simulink model "ControlDes"  (R2026a)
settings: Solver=ode3  StopTime=4  FixedStep=0.001  EnableMultiTasking=on
(part 12 of 12)

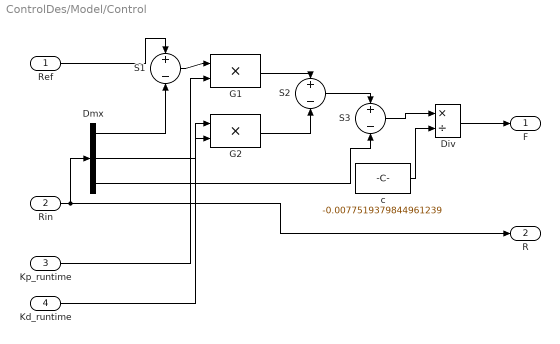
== system ControlDes/Model/Control ==
  Ref : Inport
  Rin : Inport  Port=2
  Kp_runtime : Inport  Port=3  OutDataTypeStr=double
  Kd_runtime : Inport  Port=4  OutDataTypeStr=double
  Div : Product  Inputs=*/
  Dmx : Demux  Outputs=3
  G1 : Product  Inputs=**
  G2 : Product  Inputs=**
  S1 : Sum  Inputs=+-
  S2 : Sum  Inputs=+-
  S3 : Sum  Inputs=+-
  c : Constant  Value=-0.0077519379844961239
  F : Outport
  R : Outport  Port=2
  wires:
  Div/1 -> F/1
  c/1 -> Div/2
  S3/1 -> Div/1
  Dmx/3 -> S3/2
  S2/1 -> S3/1
  G2/1 -> S2/2
  G1/1 -> S2/1
  Dmx/2 -> G2/1
  S1/1 -> G1/1
  Dmx/1 -> S1/2
  Rin/1 -> R/1, Dmx/1
  Ref/1 -> S1/1
  Kp_runtime/1 -> G1/2
  Kd_runtime/1 -> G2/2

== system ControlDes/Model/Matriz ==
  u : Inport
  A_eso_runtime : Inport  Port=2  OutDataTypeStr=double  PortDimensions=[3 3]
  B_eso_runtime : Inport  Port=3  OutDataTypeStr=double  PortDimensions=[3 2]
  C_eso_runtime : Inport  Port=4  OutDataTypeStr=double  PortDimensions=[3 3]
  D_eso_runtime : Inport  Port=5  OutDataTypeStr=double  PortDimensions=[3 2]
  A : Product  Inputs=**  Multiplication=Matrix(*)
  B : Product  Inputs=**  Multiplication=Matrix(*)
  C : Product  Inputs=**  Multiplication=Matrix(*)
  D : Product  Inputs=**  Multiplication=Matrix(*)
  State : UnitDelay  InitialCondition=[0.009;0;0]  SampleTime=0.001
  SumX : Sum
  SumY : Sum
  y : Outport
  wires:
  SumY/1 -> y/1
  D/1 -> SumY/2
  C/1 -> SumY/1
  State/1 -> A/2, C/2
  SumX/1 -> State/1
  B/1 -> SumX/2
  A/1 -> SumX/1
  u/1 -> B/2, D/2
  A_eso_runtime/1 -> A/1
  B_eso_runtime/1 -> B/1
  C_eso_runtime/1 -> C/1
  D_eso_runtime/1 -> D/1

== system ControlDes/Model1/Control ==
  Ref : Inport
  Rin : Inport  Port=2
  Kp_runtime : Inport  Port=3  OutDataTypeStr=double
  Kd_runtime : Inport  Port=4  OutDataTypeStr=double
  Div : Product  Inputs=*/
  Dmx : Demux  Outputs=3
  G1 : Product  Inputs=**
  G2 : Product  Inputs=**
  S1 : Sum  Inputs=+-
  S2 : Sum  Inputs=+-
  S3 : Sum  Inputs=+-
  c : Constant  Value=-0.010335917312661499
  F : Outport
  R : Outport  Port=2
  wires:
  Div/1 -> F/1
  c/1 -> Div/2
  S3/1 -> Div/1
  Dmx/3 -> S3/2
  S2/1 -> S3/1
  G2/1 -> S2/2
  G1/1 -> S2/1
  Dmx/2 -> G2/1
  S1/1 -> G1/1
  Dmx/1 -> S1/2
  Rin/1 -> R/1, Dmx/1
  Ref/1 -> S1/1
  Kp_runtime/1 -> G1/2
  Kd_runtime/1 -> G2/2

== system ControlDes/Model1/Matriz ==
  u : Inport
  A_eso_runtime : Inport  Port=2  OutDataTypeStr=double  PortDimensions=[3 3]
  B_eso_runtime : Inport  Port=3  OutDataTypeStr=double  PortDimensions=[3 2]
  C_eso_runtime : Inport  Port=4  OutDataTypeStr=double  PortDimensions=[3 3]
  D_eso_runtime : Inport  Port=5  OutDataTypeStr=double  PortDimensions=[3 2]
  A : Product  Inputs=**  Multiplication=Matrix(*)
  B : Product  Inputs=**  Multiplication=Matrix(*)
  C : Product  Inputs=**  Multiplication=Matrix(*)
  D : Product  Inputs=**  Multiplication=Matrix(*)
  State : UnitDelay  InitialCondition=[0.018;0;9.8]  SampleTime=0.001
  SumX : Sum
  SumY : Sum
  y : Outport
  wires:
  SumY/1 -> y/1
  D/1 -> SumY/2
  C/1 -> SumY/1
  State/1 -> A/2, C/2
  SumX/1 -> State/1
  B/1 -> SumX/2
  A/1 -> SumX/1
  u/1 -> B/2, D/2
  A_eso_runtime/1 -> A/1
  B_eso_runtime/1 -> B/1
  C_eso_runtime/1 -> C/1
  D_eso_runtime/1 -> D/1

== system ControlDes/Model2/Control ==
  Ref : Inport
  Rin : Inport  Port=2
  Kp_runtime : Inport  Port=3  OutDataTypeStr=double
  Kd_runtime : Inport  Port=4  OutDataTypeStr=double
  Div : Product  Inputs=*/
  Dmx : Demux  Outputs=3
  G1 : Product  Inputs=**
  G2 : Product  Inputs=**
  S1 : Sum  Inputs=+-
  S2 : Sum  Inputs=+-
  S3 : Sum  Inputs=+-
  c : Constant  Value=-0.010335917312661499
  F : Outport
  R : Outport  Port=2
  wires:
  Div/1 -> F/1
  c/1 -> Div/2
  S3/1 -> Div/1
  Dmx/3 -> S3/2
  S2/1 -> S3/1
  G2/1 -> S2/2
  G1/1 -> S2/1
  Dmx/2 -> G2/1
  S1/1 -> G1/1
  Dmx/1 -> S1/2
  Rin/1 -> R/1, Dmx/1
  Ref/1 -> S1/1
  Kp_runtime/1 -> G1/2
  Kd_runtime/1 -> G2/2

== system ControlDes/Model2/Matriz ==
  u : Inport
  A_eso_runtime : Inport  Port=2  OutDataTypeStr=double  PortDimensions=[3 3]
  B_eso_runtime : Inport  Port=3  OutDataTypeStr=double  PortDimensions=[3 2]
  C_eso_runtime : Inport  Port=4  OutDataTypeStr=double  PortDimensions=[3 3]
  D_eso_runtime : Inport  Port=5  OutDataTypeStr=double  PortDimensions=[3 2]
  A : Product  Inputs=**  Multiplication=Matrix(*)
  B : Product  Inputs=**  Multiplication=Matrix(*)
  C : Product  Inputs=**  Multiplication=Matrix(*)
  D : Product  Inputs=**  Multiplication=Matrix(*)
  State : UnitDelay  InitialCondition=[0.018;0;9.8]  SampleTime=0.001
  SumX : Sum
  SumY : Sum
  y : Outport
  wires:
  SumY/1 -> y/1
  D/1 -> SumY/2
  C/1 -> SumY/1
  State/1 -> A/2, C/2
  SumX/1 -> State/1
  B/1 -> SumX/2
  A/1 -> SumX/1
  u/1 -> B/2, D/2
  A_eso_runtime/1 -> A/1
  B_eso_runtime/1 -> B/1
  C_eso_runtime/1 -> C/1
  D_eso_runtime/1 -> D/1

== system ControlDes/Model3/Control ==
  Ref : Inport
  Rin : Inport  Port=2
  Kp_runtime : Inport  Port=3  OutDataTypeStr=double
  Kd_runtime : Inport  Port=4  OutDataTypeStr=double
  Div : Product  Inputs=*/
  Dmx : Demux  Outputs=3
  G1 : Product  Inputs=**
  G2 : Product  Inputs=**
  S1 : Sum  Inputs=+-
  S2 : Sum  Inputs=+-
  S3 : Sum  Inputs=+-
  c : Constant  Value=-0.010335917312661499
  F : Outport
  wires:
  Div/1 -> F/1
  c/1 -> Div/2
  S3/1 -> Div/1
  Dmx/3 -> S3/2
  S2/1 -> S3/1
  G2/1 -> S2/2
  G1/1 -> S2/1
  Dmx/2 -> G2/1
  S1/1 -> G1/1
  Dmx/1 -> S1/2
  Rin/1 -> Dmx/1
  Ref/1 -> S1/1
  Kp_runtime/1 -> G1/2
  Kd_runtime/1 -> G2/2

== system ControlDes/Model3/Matriz ==
  u : Inport
  A_eso_runtime : Inport  Port=2  OutDataTypeStr=double  PortDimensions=[3 3]
  B_eso_runtime : Inport  Port=3  OutDataTypeStr=double  PortDimensions=[3 2]
  C_eso_runtime : Inport  Port=4  OutDataTypeStr=double  PortDimensions=[3 3]
  D_eso_runtime : Inport  Port=5  OutDataTypeStr=double  PortDimensions=[3 2]
  A : Product  Inputs=**  Multiplication=Matrix(*)
  B : Product  Inputs=**  Multiplication=Matrix(*)
  C : Product  Inputs=**  Multiplication=Matrix(*)
  D : Product  Inputs=**  Multiplication=Matrix(*)
  State : UnitDelay  InitialCondition=[0.018;0;9.8]  SampleTime=0.001
  SumX : Sum
  SumY : Sum
  y : Outport
  wires:
  SumY/1 -> y/1
  D/1 -> SumY/2
  C/1 -> SumY/1
  State/1 -> A/2, C/2
  SumX/1 -> State/1
  B/1 -> SumX/2
  A/1 -> SumX/1
  u/1 -> B/2, D/2
  A_eso_runtime/1 -> A/1
  B_eso_runtime/1 -> B/1
  C_eso_runtime/1 -> C/1
  D_eso_runtime/1 -> D/1

== system ControlDes/Model4/Control ==
  Ref : Inport
  Rin : Inport  Port=2
  Kp_runtime : Inport  Port=3  OutDataTypeStr=double
  Kd_runtime : Inport  Port=4  OutDataTypeStr=double
  Div : Product  Inputs=*/
  Dmx : Demux  Outputs=3
  G1 : Product  Inputs=**
  G2 : Product  Inputs=**
  S1 : Sum  Inputs=+-
  S2 : Sum  Inputs=+-
  S3 : Sum  Inputs=+-
  c : Constant  Value=-0.0077519379844961239
  F : Outport
  R : Outport  Port=2
  wires:
  Div/1 -> F/1
  c/1 -> Div/2
  S3/1 -> Div/1
  Dmx/3 -> S3/2
  S2/1 -> S3/1
  G2/1 -> S2/2
  G1/1 -> S2/1
  Dmx/2 -> G2/1
  S1/1 -> G1/1
  Dmx/1 -> S1/2
  Rin/1 -> R/1, Dmx/1
  Ref/1 -> S1/1
  Kp_runtime/1 -> G1/2
  Kd_runtime/1 -> G2/2

== system ControlDes/Model4/Matriz ==
  u : Inport
  A_eso_runtime : Inport  Port=2  OutDataTypeStr=double  PortDimensions=[3 3]
  B_eso_runtime : Inport  Port=3  OutDataTypeStr=double  PortDimensions=[3 2]
  C_eso_runtime : Inport  Port=4  OutDataTypeStr=double  PortDimensions=[3 3]
  D_eso_runtime : Inport  Port=5  OutDataTypeStr=double  PortDimensions=[3 2]
  A : Product  Inputs=**  Multiplication=Matrix(*)
  B : Product  Inputs=**  Multiplication=Matrix(*)
  C : Product  Inputs=**  Multiplication=Matrix(*)
  D : Product  Inputs=**  Multiplication=Matrix(*)
  State : UnitDelay  InitialCondition=[0.01023;0;0]  SampleTime=0.001
  SumX : Sum
  SumY : Sum
  y : Outport
  wires:
  SumY/1 -> y/1
  D/1 -> SumY/2
  C/1 -> SumY/1
  State/1 -> A/2, C/2
  SumX/1 -> State/1
  B/1 -> SumX/2
  A/1 -> SumX/1
  u/1 -> B/2, D/2
  A_eso_runtime/1 -> A/1
  B_eso_runtime/1 -> B/1
  C_eso_runtime/1 -> C/1
  D_eso_runtime/1 -> D/1

== system ControlDes/Model5/Control ==
  Ref : Inport
  Rin : Inport  Port=2
  Kp_runtime : Inport  Port=3  OutDataTypeStr=double
  Kd_runtime : Inport  Port=4  OutDataTypeStr=double
  Div : Product  Inputs=*/
  Dmx : Demux  Outputs=3
  G1 : Product  Inputs=**
  G2 : Product  Inputs=**
  S1 : Sum  Inputs=+-
  S2 : Sum  Inputs=+-
  S3 : Sum  Inputs=+-
  c : Constant  Value=-0.010335917312661499
  F : Outport
  R : Outport  Port=2
  wires:
  Div/1 -> F/1
  c/1 -> Div/2
  S3/1 -> Div/1
  Dmx/3 -> S3/2
  S2/1 -> S3/1
  G2/1 -> S2/2
  G1/1 -> S2/1
  Dmx/2 -> G2/1
  S1/1 -> G1/1
  Dmx/1 -> S1/2
  Rin/1 -> R/1, Dmx/1
  Ref/1 -> S1/1
  Kp_runtime/1 -> G1/2
  Kd_runtime/1 -> G2/2

== system ControlDes/Model5/Matriz ==
  u : Inport
  A_eso_runtime : Inport  Port=2  OutDataTypeStr=double  PortDimensions=[3 3]
  B_eso_runtime : Inport  Port=3  OutDataTypeStr=double  PortDimensions=[3 2]
  C_eso_runtime : Inport  Port=4  OutDataTypeStr=double  PortDimensions=[3 3]
  D_eso_runtime : Inport  Port=5  OutDataTypeStr=double  PortDimensions=[3 2]
  A : Product  Inputs=**  Multiplication=Matrix(*)
  B : Product  Inputs=**  Multiplication=Matrix(*)
  C : Product  Inputs=**  Multiplication=Matrix(*)
  D : Product  Inputs=**  Multiplication=Matrix(*)
  State : UnitDelay  InitialCondition=[0.018;0;9.8]  SampleTime=0.001
  SumX : Sum
  SumY : Sum
  y : Outport
  wires:
  SumY/1 -> y/1
  D/1 -> SumY/2
  C/1 -> SumY/1
  State/1 -> A/2, C/2
  SumX/1 -> State/1
  B/1 -> SumX/2
  A/1 -> SumX/1
  u/1 -> B/2, D/2
  A_eso_runtime/1 -> A/1
  B_eso_runtime/1 -> B/1
  C_eso_runtime/1 -> C/1
  D_eso_runtime/1 -> D/1

== system ControlDes/Model6/Control ==
  Ref : Inport
  Rin : Inport  Port=2
  Kp_runtime : Inport  Port=3  OutDataTypeStr=double
  Kd_runtime : Inport  Port=4  OutDataTypeStr=double
  Div : Product  Inputs=*/
  Dmx : Demux  Outputs=3
  G1 : Product  Inputs=**
  G2 : Product  Inputs=**
  S1 : Sum  Inputs=+-
  S2 : Sum  Inputs=+-
  S3 : Sum  Inputs=+-
  c : Constant  Value=-0.0077519379844961239
  F : Outport
  R : Outport  Port=2
  wires:
  Div/1 -> F/1
  c/1 -> Div/2
  S3/1 -> Div/1
  Dmx/3 -> S3/2
  S2/1 -> S3/1
  G2/1 -> S2/2
  G1/1 -> S2/1
  Dmx/2 -> G2/1
  S1/1 -> G1/1
  Dmx/1 -> S1/2
  Rin/1 -> R/1, Dmx/1
  Ref/1 -> S1/1
  Kp_runtime/1 -> G1/2
  Kd_runtime/1 -> G2/2

== system ControlDes/Model6/Matriz ==
  u : Inport
  A_eso_runtime : Inport  Port=2  OutDataTypeStr=double  PortDimensions=[3 3]
  B_eso_runtime : Inport  Port=3  OutDataTypeStr=double  PortDimensions=[3 2]
  C_eso_runtime : Inport  Port=4  OutDataTypeStr=double  PortDimensions=[3 3]
  D_eso_runtime : Inport  Port=5  OutDataTypeStr=double  PortDimensions=[3 2]
  A : Product  Inputs=**  Multiplication=Matrix(*)
  B : Product  Inputs=**  Multiplication=Matrix(*)
  C : Product  Inputs=**  Multiplication=Matrix(*)
  D : Product  Inputs=**  Multiplication=Matrix(*)
  State : UnitDelay  InitialCondition=[0.009;0;0]  SampleTime=0.001
  SumX : Sum
  SumY : Sum
  y : Outport
  wires:
  SumY/1 -> y/1
  D/1 -> SumY/2
  C/1 -> SumY/1
  State/1 -> A/2, C/2
  SumX/1 -> State/1
  B/1 -> SumX/2
  A/1 -> SumX/1
  u/1 -> B/2, D/2
  A_eso_runtime/1 -> A/1
  B_eso_runtime/1 -> B/1
  C_eso_runtime/1 -> C/1
  D_eso_runtime/1 -> D/1

== system ControlDes/Model7/Control ==
  Ref : Inport
  Rin : Inport  Port=2
  Kp_runtime : Inport  Port=3  OutDataTypeStr=double
  Kd_runtime : Inport  Port=4  OutDataTypeStr=double
  Div : Product  Inputs=*/
  Dmx : Demux  Outputs=3
  G1 : Product  Inputs=**
  G2 : Product  Inputs=**
  S1 : Sum  Inputs=+-
  S2 : Sum  Inputs=+-
  S3 : Sum  Inputs=+-
  c : Constant  Value=-0.0077519379844961239
  F : Outport
  R : Outport  Port=2
  wires:
  Div/1 -> F/1
  c/1 -> Div/2
  S3/1 -> Div/1
  Dmx/3 -> S3/2
  S2/1 -> S3/1
  G2/1 -> S2/2
  G1/1 -> S2/1
  Dmx/2 -> G2/1
  S1/1 -> G1/1
  Dmx/1 -> S1/2
  Rin/1 -> R/1, Dmx/1
  Ref/1 -> S1/1
  Kp_runtime/1 -> G1/2
  Kd_runtime/1 -> G2/2

== system ControlDes/Model7/Matriz ==
  u : Inport
  A_eso_runtime : Inport  Port=2  OutDataTypeStr=double  PortDimensions=[3 3]
  B_eso_runtime : Inport  Port=3  OutDataTypeStr=double  PortDimensions=[3 2]
  C_eso_runtime : Inport  Port=4  OutDataTypeStr=double  PortDimensions=[3 3]
  D_eso_runtime : Inport  Port=5  OutDataTypeStr=double  PortDimensions=[3 2]
  A : Product  Inputs=**  Multiplication=Matrix(*)
  B : Product  Inputs=**  Multiplication=Matrix(*)
  C : Product  Inputs=**  Multiplication=Matrix(*)
  D : Product  Inputs=**  Multiplication=Matrix(*)
  State : UnitDelay  InitialCondition=[0.01023;0;0]  SampleTime=0.001
  SumX : Sum
  SumY : Sum
  y : Outport
  wires:
  SumY/1 -> y/1
  D/1 -> SumY/2
  C/1 -> SumY/1
  State/1 -> A/2, C/2
  SumX/1 -> State/1
  B/1 -> SumX/2
  A/1 -> SumX/1
  u/1 -> B/2, D/2
  A_eso_runtime/1 -> A/1
  B_eso_runtime/1 -> B/1
  C_eso_runtime/1 -> C/1
  D_eso_runtime/1 -> D/1

== system ControlDes/Model8/Control ==
  Ref : Inport
  Rin : Inport  Port=2
  Kp_runtime : Inport  Port=3  OutDataTypeStr=double
  Kd_runtime : Inport  Port=4  OutDataTypeStr=double
  Div : Product  Inputs=*/
  Dmx : Demux  Outputs=3
  G1 : Product  Inputs=**
  G2 : Product  Inputs=**
  S1 : Sum  Inputs=+-
  S2 : Sum  Inputs=+-
  S3 : Sum  Inputs=+-
  c : Constant  Value=-0.0077519379844961239
  F : Outport
  R : Outport  Port=2
  wires:
  Div/1 -> F/1
  c/1 -> Div/2
  S3/1 -> Div/1
  Dmx/3 -> S3/2
  S2/1 -> S3/1
  G2/1 -> S2/2
  G1/1 -> S2/1
  Dmx/2 -> G2/1
  S1/1 -> G1/1
  Dmx/1 -> S1/2
  Rin/1 -> R/1, Dmx/1
  Ref/1 -> S1/1
  Kp_runtime/1 -> G1/2
  Kd_runtime/1 -> G2/2

== system ControlDes/Model8/Matriz ==
  u : Inport
  A_eso_runtime : Inport  Port=2  OutDataTypeStr=double  PortDimensions=[3 3]
  B_eso_runtime : Inport  Port=3  OutDataTypeStr=double  PortDimensions=[3 2]
  C_eso_runtime : Inport  Port=4  OutDataTypeStr=double  PortDimensions=[3 3]
  D_eso_runtime : Inport  Port=5  OutDataTypeStr=double  PortDimensions=[3 2]
  A : Product  Inputs=**  Multiplication=Matrix(*)
  B : Product  Inputs=**  Multiplication=Matrix(*)
  C : Product  Inputs=**  Multiplication=Matrix(*)
  D : Product  Inputs=**  Multiplication=Matrix(*)
  State : UnitDelay  InitialCondition=[0.009;0;0]  SampleTime=0.001
  SumX : Sum
  SumY : Sum
  y : Outport
  wires:
  SumY/1 -> y/1
  D/1 -> SumY/2
  C/1 -> SumY/1
  State/1 -> A/2, C/2
  SumX/1 -> State/1
  B/1 -> SumX/2
  A/1 -> SumX/1
  u/1 -> B/2, D/2
  A_eso_runtime/1 -> A/1
  B_eso_runtime/1 -> B/1
  C_eso_runtime/1 -> C/1
  D_eso_runtime/1 -> D/1

== system ControlDes/Model9/Control ==
  Ref : Inport
  Rin : Inport  Port=2
  Kp_runtime : Inport  Port=3  OutDataTypeStr=double
  Kd_runtime : Inport  Port=4  OutDataTypeStr=double
  Div : Product  Inputs=*/
  Dmx : Demux  Outputs=3
  G1 : Product  Inputs=**
  G2 : Product  Inputs=**
  S1 : Sum  Inputs=+-
  S2 : Sum  Inputs=+-
  S3 : Sum  Inputs=+-
  c : Constant  Value=-0.0077519379844961239
  F : Outport
  R : Outport  Port=2
  wires:
  Div/1 -> F/1
  c/1 -> Div/2
  S3/1 -> Div/1
  Dmx/3 -> S3/2
  S2/1 -> S3/1
  G2/1 -> S2/2
  G1/1 -> S2/1
  Dmx/2 -> G2/1
  S1/1 -> G1/1
  Dmx/1 -> S1/2
  Rin/1 -> R/1, Dmx/1
  Ref/1 -> S1/1
  Kp_runtime/1 -> G1/2
  Kd_runtime/1 -> G2/2

== system ControlDes/Model9/Matriz ==
  u : Inport
  A_eso_runtime : Inport  Port=2  OutDataTypeStr=double  PortDimensions=[3 3]
  B_eso_runtime : Inport  Port=3  OutDataTypeStr=double  PortDimensions=[3 2]
  C_eso_runtime : Inport  Port=4  OutDataTypeStr=double  PortDimensions=[3 3]
  D_eso_runtime : Inport  Port=5  OutDataTypeStr=double  PortDimensions=[3 2]
  A : Product  Inputs=**  Multiplication=Matrix(*)
  B : Product  Inputs=**  Multiplication=Matrix(*)
  C : Product  Inputs=**  Multiplication=Matrix(*)
  D : Product  Inputs=**  Multiplication=Matrix(*)
  State : UnitDelay  InitialCondition=[0.01023;0;0]  SampleTime=0.001
  SumX : Sum
  SumY : Sum
  y : Outport
  wires:
  SumY/1 -> y/1
  D/1 -> SumY/2
  C/1 -> SumY/1
  State/1 -> A/2, C/2
  SumX/1 -> State/1
  B/1 -> SumX/2
  A/1 -> SumX/1
  u/1 -> B/2, D/2
  A_eso_runtime/1 -> A/1
  B_eso_runtime/1 -> B/1
  C_eso_runtime/1 -> C/1
  D_eso_runtime/1 -> D/1

== matlab function ControlDes/Model2/MATLAB Function6 ==
  data: x input; y output
function y = notch_filter(x)
%#codegen
% z 20.305 Hz
Ts=0.001;
persistent x1 x2 y1 y2 b0 b1 b2 a1 a2 init
if isempty(init)
    [b0,b1,b2,a1,a2]=coef(20.30544132864105,2,Ts);x1=x;x2=x;y1=x;y2=x;init=true;
end
y=b0*x+b1*x1+b2*x2-a1*y1-a2*y2;x2=x1;x1=x;y2=y1;y1=y;
end
function [b0,b1,b2,a1,a2]=coef(f,bw,Ts)
w=2*pi*f;Q=f/bw;c=2/Ts;d=c^2+(w/Q)*c+w^2;b0=(c^2+w^2)/d;b1=(-2*c^2+2*w^2)/d;b2=b0;a1=b1;a2=(c^2-(w/Q)*c+w^2)/d;
end

== matlab function ControlDes/Model1/MATLAB Function6 ==
  data: x input; y output
function y = notch_filter(x)
%#codegen
% z 20.305 Hz
Ts=0.001;
persistent x1 x2 y1 y2 b0 b1 b2 a1 a2 init
if isempty(init)
    [b0,b1,b2,a1,a2]=coef(20.30544132864105,2,Ts);x1=x;x2=x;y1=x;y2=x;init=true;
end
y=b0*x+b1*x1+b2*x2-a1*y1-a2*y2;x2=x1;x1=x;y2=y1;y1=y;
end
function [b0,b1,b2,a1,a2]=coef(f,bw,Ts)
w=2*pi*f;Q=f/bw;c=2/Ts;d=c^2+(w/Q)*c+w^2;b0=(c^2+w^2)/d;b1=(-2*c^2+2*w^2)/d;b2=b0;a1=b1;a2=(c^2-(w/Q)*c+w^2)/d;
end

== matlab function ControlDes/Model5/MATLAB Function6 ==
  data: x input; y output
function y = notch_filter(x)
%#codegen
% z 20.305 Hz
Ts=0.001;
persistent x1 x2 y1 y2 b0 b1 b2 a1 a2 init
if isempty(init)
    [b0,b1,b2,a1,a2]=coef(20.30544132864105,2,Ts);x1=x;x2=x;y1=x;y2=x;init=true;
end
y=b0*x+b1*x1+b2*x2-a1*y1-a2*y2;x2=x1;x1=x;y2=y1;y1=y;
end
function [b0,b1,b2,a1,a2]=coef(f,bw,Ts)
w=2*pi*f;Q=f/bw;c=2/Ts;d=c^2+(w/Q)*c+w^2;b0=(c^2+w^2)/d;b1=(-2*c^2+2*w^2)/d;b2=b0;a1=b1;a2=(c^2-(w/Q)*c+w^2)/d;
end

== matlab function ControlDes/SensorSpaceNotch20p94 ==
  data: gaps input; gaps_out output
function gaps_out = sensor_space_notch(gaps)
%#codegen
Ts = 0.001;
f = 20.939691191057825;
bw = 4.0;
persistent x1 x2 y1 y2 initialized
if isempty(initialized)
    x1=zeros(4,1);x2=zeros(4,1);y1=zeros(4,1);y2=zeros(4,1);
    for i=1:4
        x1(i)=gaps(i);x2(i)=gaps(i);
        y1(i)=gaps(i);y2(i)=gaps(i);
    end
    initialized=true;
end
w=2*pi*f;Q=f/bw;c=2/Ts;d=c*c+(w/Q)*c+w*w;
b0=(c*c+w*w)/d;
b1=(-2*c*c+2*w*w)/d;
b2=b0;a1=b1;a2=(c*c-(w/Q)*c+w*w)/d;
gaps_out=gaps;
for i=1:4
    y=b0*gaps(i)+b1*x1(i)+b2*x2(i)-a1*y1(i)-a2*y2(i);
    x2(i)=x1(i);x1(i)=gaps(i);y2(i)=y1(i);y1(i)=y;
    gaps_out(i)=y;
end
end

== matlab function ControlDes/Model3/MATLAB Function6 ==
  data: x input; y output
function y = notch_filter(x)
%#codegen
% z 20.305 Hz
Ts=0.001;
persistent x1 x2 y1 y2 b0 b1 b2 a1 a2 init
if isempty(init)
    [b0,b1,b2,a1,a2]=coef(20.30544132864105,2,Ts);x1=x;x2=x;y1=x;y2=x;init=true;
end
y=b0*x+b1*x1+b2*x2-a1*y1-a2*y2;x2=x1;x1=x;y2=y1;y1=y;
end
function [b0,b1,b2,a1,a2]=coef(f,bw,Ts)
w=2*pi*f;Q=f/bw;c=2/Ts;d=c^2+(w/Q)*c+w^2;b0=(c^2+w^2)/d;b1=(-2*c^2+2*w^2)/d;b2=b0;a1=b1;a2=(c^2-(w/Q)*c+w^2)/d;
end

== matlab function ControlDes/MATLAB Function1 ==
  data: posicion input; airgaps_actuadores output
function airgaps_actuadores = GapsLocales(posicion)

%#codegen

    y = posicion(1);
    z = posicion(2);
    rotx = posicion(3);
    roty = posicion(4);
    rotz = posicion(5);

    %% Actuadores HEMS desde CG
    % Datos.m -> ph. Orden: [DI; DD; TI; TD]. Columnas: [x y z] en metros.
    hems_pos = [ ...
         0.93085, -0.27376, 0.09316; ...
         0.93085,  0.27124, 0.09316; ...
        -0.96315, -0.27376, 0.09316; ...
        -0.96315,  0.27124, 0.09316];

    x_h = hems_pos(:,1);
    y_h = hems_pos(:,2);

    g_h = abs(z + y_h.*sin(rotx) - x_h.*sin(roty));

    AG1 = g_h(1); 
    AG2 = g_h(2);  
    AG3 = g_h(3); 
    AG4 = g_h(4);  

    %% Actuadores EMS desde CG
    % Datos.m -> pe. Orden: [DI; DD; CI; CD; TI; TD].
    ems_pos = [ ...
         0.75185, -0.35003, 0.22816; ...
         0.75185,  0.34674, 0.22816; ...
        -0.01615, -0.35003, 0.22816; ...
        -0.01615,  0.34674, 0.22816; ...
        -0.78415, -0.35003, 0.22818; ...
        -0.78415,  0.34674, 0.22816];

    x_e = ems_pos(:,1);
    y_e = ems_pos(:,2);
    z_e = ems_pos(:,3);
    y_rail_left = -0.35903;
    y_rail_right = 0.35697;

    side_e = [-1; 1; -1; 1; -1; 1];
    rail_e = [y_rail_left; y_rail_right; ...
              y_rail_left; y_rail_right; ...
              y_rail_left; y_rail_right];

    r_y = y_e.*cos(rotz) ...
          + x_e.*sin(rotz) ...
          - z_e.*sin(rotx);

    g_e = abs(side_e.*(rail_e - r_y - y));

    AG5 = g_e(1);   
    AG6 = g_e(2);   
    AG7 = g_e(3);   
    AG8 = g_e(4);   
    AG9 = g_e(5);   
    AG10 = g_e(6);  

    airgaps_actuadores = [AG1; AG2; AG3; AG4; AG5; AG6; AG7; AG8; AG9; AG10];
end

== matlab function ControlDes/GapToStates ==
  data: airgaps input; u output
function u = Sensores_A_Estados(airgaps)
%#codegen

    ag1 = airgaps(1);
    ag2 = airgaps(2);
    ag3 = airgaps(3);
    ag4 = airgaps(4);
    ag5 = airgaps(5);
    ag6 = airgaps(6);
    ag7 = airgaps(7);
    ag8 = airgaps(8);

    %% Constantes generales
    t_via = 0.015;         
    z_HEMS_CG = 0.0932;     
    L_der = 356.97e-3;      
    L_iz  = 359.03e-3;      

    %% Sensores verticales
    % Orden: izquierdo delantero, derecho delantero, izquierdo trasero,
    % derecho trasero. Columnas: [x y z] en metros.
    sensores_v = [ ...
         1.21436, -0.31280, -0.00782; ...
         1.21636,  0.31027, -0.00782; ...
        -1.24866, -0.31280, -0.00782; ...
        -1.24666,  0.31027, -0.00782];

    x_v = sensores_v(:,1);
    y_v = sensores_v(:,2);
    z_v = sensores_v(:,3);

    g_v = [ag1; ag2; ag3; ag4];

    b_v = -g_v - t_via + z_HEMS_CG - z_v;
    H_v = [ones(4,1), y_v, -x_v];

    theta_v = H_v \ b_v;

    rotx = theta_v(2);
    roty = theta_v(3);

    z_aux = -g_v ...
            - t_via ...
            + z_HEMS_CG ...
            - z_v.*cos(rotx) ...
            + x_v.*sin(roty) ...
            - y_v.*sin(rotx);

    z = mean(z_aux);

    %% Sensores laterales
    % Orden: izquierdo delantero, derecho delantero, izquierdo trasero,
    % derecho trasero. Columnas: [x y z] en metros.
    sensores_l = [ ...
         1.24634, -0.28497, 0.26891; ...
         1.24834,  0.28244, 0.26891; ...
        -1.28064, -0.28497, 0.26891; ...
        -1.27864,  0.28244, 0.26891];

    x_l = sensores_l(:,1);
    y_l = sensores_l(:,2);
    z_l = sensores_l(:,3);  

   
    side_l = [-1; 1; -1; 1];
    y_rail_l = [-L_iz; L_der; -L_iz; L_der];

    g_l = [ag5; ag6; ag7; ag8];

    b_l = y_rail_l - side_l.*g_l + z_l.*sin(rotx);
    H_l = [ones(4,1), y_l, x_l];

    theta_l = H_l \ b_l;

    cos_rotz = theta_l(2);
    sin_rotz = theta_l(3);
    rotz = atan2(sin_rotz, cos_rotz);

    r_y = y_l.*cos(rotz) ...
          + x_l.*sin(rotz) ...
          - z_l.*sin(rotx);

    y_aux = y_rail_l - side_l.*g_l - r_y;
    y = mean(y_aux);

    u = [y; z; rotx; roty; rotz];
end
